simulink model "Comparison_Systems_Hybrid"  (R2017a)
settings: Solver=ode4  StartTime=0.0  StopTime=0.1  FixedStep=Tsim  RelTol=1e-3
values from neighbouring files (symbols this model uses):
  a = 25    [Stetup_HIL.m]
  K = 20    [Stetup_HIL.m]
  T = 1/Fs    (= 0.002)    [Stetup_HIL.m]
  zg = K*(1-exp(-a*T))    [Stetup_HIL.m]
  zp = exp(-a*T)    [Stetup_HIL.m]
settings Model: Creator=tac29  LastModifiedBy=Merc

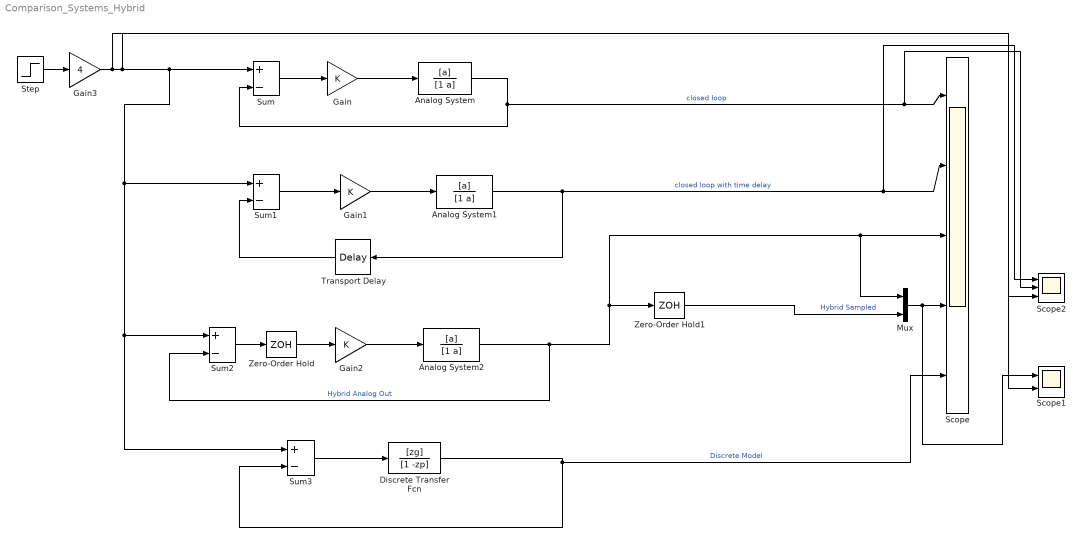
== system Comparison_Systems_Hybrid ==
  Analog System : TransferFcn  Numerator=[a]  Denominator=[1 a]
  Analog System1 : TransferFcn  Numerator=[a]  Denominator=[1 a]
  Analog System2 : TransferFcn  Numerator=[a]  Denominator=[1 a]
  Discrete Transfer Fcn : DiscreteTransferFcn  Numerator=[zg]  Denominator=[1 -zp]  SampleTime=T
  Gain : Gain  Gain=K
  Gain1 : Gain  Gain=K
  Gain2 : Gain  Gain=K
  Gain3 : Gain  Gain=4
  Mux : Mux  Inputs=2
  Scope : Scope  NumInputPorts=5
  Scope1 : Scope  NumInputPorts=2
  Scope2 : Scope  NumInputPorts=3
  Step : Step  Time=.01  SampleTime=0
  Sum{,1..3} (4 alike) : Sum  Inputs=+-
  Transport Delay : TransportDelay  DelayTime=T
  Zero-Order Hold : ZeroOrderHold  SampleTime=T
  Zero-Order Hold1 : ZeroOrderHold  SampleTime=T
  wires:
  Analog System/1 -> Scope2/2, Scope/1, Sum/2  "closed loop"
  Sum/1 -> Gain/1
  Gain/1 -> Analog System/1
  Step/1 -> Gain3/1
  Sum1/1 -> Gain1/1
  Gain1/1 -> Analog System1/1
  Analog System1/1 -> Transport Delay/1, Scope2/1, Scope/2  "closed loop with time delay"
  Transport Delay/1 -> Sum1/2
  Analog System2/1 -> Sum2/2, Mux/1, Scope/3, Zero-Order Hold1/1  "Hybrid Analog Out"
  Gain2/1 -> Analog System2/1
  Sum2/1 -> Zero-Order Hold/1
  Zero-Order Hold/1 -> Gain2/1
  Sum3/1 -> Discrete Transfer Fcn/1
  Discrete Transfer Fcn/1 -> Sum3/2, Scope/5  "Discrete Model"
  Gain3/1 -> Scope2/3, Scope1/2, Sum1/1, Sum3/1, Sum2/1, Sum/1
  Zero-Order Hold1/1 -> Mux/2  "Hybrid Sampled"
  Mux/1 -> Scope1/1, Scope/4
